simulink model "nonlinear_closed_g"  (R2024a)
settings: Solver=VariableStepAuto  StartTime=0.0  StopTime=30  MaxStep=1e-3  RelTol=1e-3
values from neighbouring files (symbols this model uses):
  A = [0, 1, 0, 0 ... (first row only)    [t_51.m]    (also in t_52.m)
  B = [0; J/Meff; 0; -beta/Meff]    [t_51.m]    (also in t_52.m)
  beta = m * lc    (= 40.0551)    [t_51.m]    (also in t_52.m)
  g = 9.81    [t_51.m]    (also in t_52.m)
  G_g = zeros(p_g)    [t_52.m]
  J = (1/3)*m1*l^2 + m2*l^2    (= 62.720658)    [t_51.m]    (also in t_52.m)
  K = [-46.28, -233.21, -10984.45, -3688.10]    [t_51.m]    (also in t_52.m)
  K_g = (U_g - K * X_g)    [t_52.m]
  M = 658.36    [t_51.m]    (also in t_52.m)
  m = m1 + m2    (= 30.46)    [t_51.m]    (also in t_52.m)
  w_g0 = zeros(p_g, 1)    [t_52.m]
  x0 = [0.1; 0.2; 0.03; 0.12]    [t_51.m]    (also in t_52.m)
  Y_g = zeros(1, p_g)    [t_52.m]
settings Model: Creator=eva  LastModifiedBy=eva

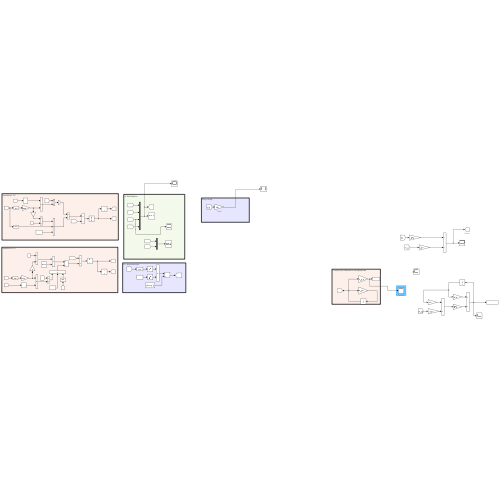
[thumbnail: Simulink's stored preview of the top-level diagram]
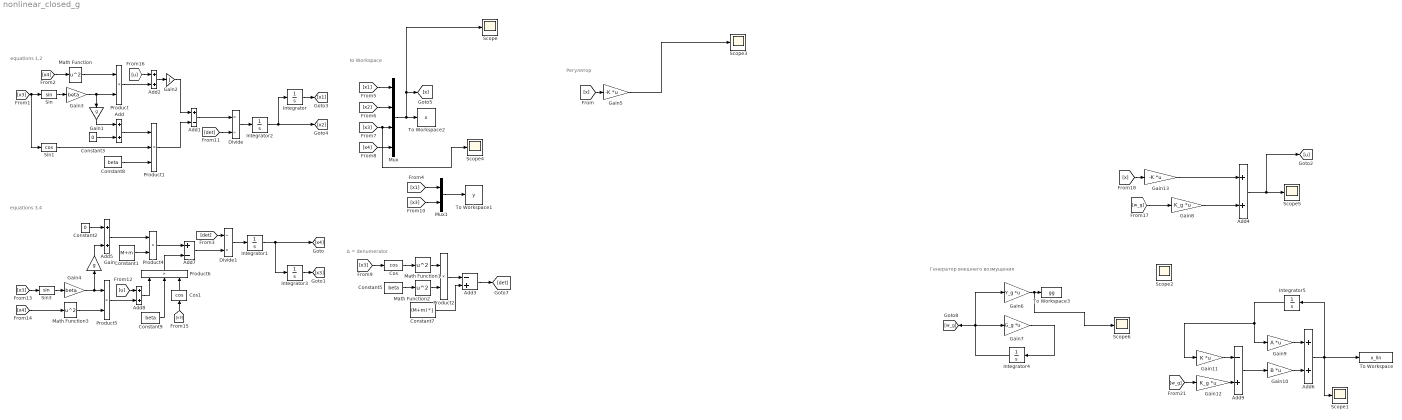
== system nonlinear_closed_g ==
  note: Регулятор
  note: to Workspace
  note: equations 1,2
  note: equations 3,4
  note: Δ = denumerator
  note: Генератор внешнего возмущения
  Add{,2,4..6,8} (6 alike) : Sum
  Add1 : Sum  Inputs=+-
  Add3 : Sum  Inputs=-+
  Add7 : Sum  Inputs=+-
  Add9 : Sum  Inputs=-+
  Constant1 : Constant  Value=M+m
  Constant2 : Constant  Value=0
  Constant3 : Constant  Value=0
  Constant5 : Constant  Value=beta
  Constant7 : Constant  Value=(M+m) * J
  Constant8 : Constant  Value=beta
  Constant9 : Constant  Value=beta
  Cos : Trigonometry  Operator=cos
  Cos1 : Trigonometry  Operator=cos
  Divide : Product  Inputs=*/
  Divide1 : Product  Inputs=/*
  Gain : Gain  Gain=g
  Gain1 : Gain  Gain=g
  Gain10 : Gain  Gain=B  Multiplication=Matrix(K*u)
  Gain11 : Gain  Gain=K  Multiplication=Matrix(K*u)
  Gain12 : Gain  Gain=K_g  Multiplication=Matrix(K*u)
  Gain13 : Gain  Gain=-K  Multiplication=Matrix(K*u)
  Gain2 : Gain  Gain=J
  Gain3 : Gain  Gain=beta
  Gain4 : Gain  Gain=beta
  Gain5 : Gain  Gain=-K  Multiplication=Matrix(K*u)
  Gain6 : Gain  Gain=Y_g  Multiplication=Matrix(K*u)
  Gain7 : Gain  Gain=G_g  Multiplication=Matrix(K*u)
  Gain8 : Gain  Gain=K_g  Multiplication=Matrix(K*u)
  Gain9 : Gain  Gain=A  Multiplication=Matrix(K*u)
  Integrator : Integrator  InitialCondition=x0(1)
  Integrator1 : Integrator  InitialCondition=x0(4)
  Integrator2 : Integrator  InitialCondition=x0(2)
  Integrator3 : Integrator  InitialCondition=x0(3)
  Integrator4 : Integrator  InitialCondition=w_g0
  Integrator5 : Integrator  InitialCondition=x0
  Math Function{,1..3} (4 alike) : Math  Operator=square
  Mux : Mux
  Mux1 : Mux  Inputs=2
  Product{,2,4..5} (4 alike) : Product
  Product1 : Product  Inputs=3
  Product6 : Product  Inputs=3
  Scope{,1..6} (7 alike) : Scope
  Sin : Trigonometry
  Sin1 : Trigonometry  Operator=cos
  Sin3 : Trigonometry
  To Workspace : ToWorkspace  VariableName=x_lin  SaveFormat=Structure With Time  SampleTime=-1
  To Workspace1 : ToWorkspace  VariableName=y  SaveFormat=Structure With Time  SampleTime=-1
  To Workspace2 : ToWorkspace  VariableName=x  SaveFormat=Structure With Time  SampleTime=-1
  To Workspace3 : ToWorkspace  VariableName=gg  SaveFormat=Structure With Time  SampleTime=-1
  wires:
  Divide/1 -> Integrator2/1
  Mux1/1 -> To Workspace1/1
  [x3] -> Mux1/2
  Gain3/1 -> Product/2, Gain1/1
  Sin/1 -> Gain3/1
  Mux/1 -> Scope/1, [x], To Workspace2/1
  Divide1/1 -> Integrator1/1
  Integrator2/1 -> [x2], Integrator/1
  Math Function3/1 -> Product5/2
  Constant8/1 -> Product1/3
  Math Function/1 -> Product/1
  [x4] -> Math Function/1
  [det] -> Divide/2
  [u] -> Add2/1
  Gain2/1 -> Add1/1
  Add/1 -> Product1/1
  [x3] -> Cos/1
  Math Function2/1 -> Product2/2
  Product4/1 -> Add7/1
  Constant3/1 -> Add/2
  Add2/1 -> Gain2/1
  [x3] -> Cos1/1
  [u] -> Add8/1
  Constant7/1 -> Add3/2
  Cos1/1 -> Product6/3
  [det] -> Divide1/1
  Constant9/1 -> Product6/2
  Math Function1/1 -> Product2/1
  [x3] -> Sin/1, Sin1/1
  [x4] -> Math Function3/1
  Product2/1 -> Add3/1
  Add8/1 -> Product6/1
  Integrator1/1 -> [x4], Integrator3/1
  Product5/1 -> Add8/2
  [x4] -> Mux/4
  [x3] -> Sin3/1
  Sin1/1 -> Product1/2
  Constant2/1 -> Add5/1
  Sin3/1 -> Gain4/1
  [x1] -> Mux/1
  Gain1/1 -> Add/1
  Gain/1 -> Add5/2
  Product6/1 -> Add7/2
  [x1] -> Mux1/1
  [x3] -> Scope4/1, Mux/3
  [x2] -> Mux/2
  Add7/1 -> Divide1/2
  Add3/1 -> [det]
  Integrator/1 -> [x1]
  Add1/1 -> Divide/1
  Product/1 -> Add2/2
  Constant5/1 -> Math Function2/1
  Gain5/1 -> Scope3/1
  Product1/1 -> Add1/2
  Gain4/1 -> Product5/1, Gain/1
  Integrator3/1 -> [x3]
  Cos/1 -> Math Function1/1
  Constant1/1 -> Product4/2
  Add5/1 -> Product4/1
  [x] -> Gain5/1
  Integrator4/1 -> [w_g], Gain7/1, Gain6/1
  [w_g] -> Gain12/1
  Gain9/1 -> Add6/1
  Gain6/1 -> Scope6/1, To Workspace3/1
  Gain10/1 -> Add6/2
  Add9/1 -> Gain10/1
  Gain12/1 -> Add9/2
  Integrator5/1 -> Gain9/1, Gain11/1
  Gain7/1 -> Integrator4/1
  [w_g] -> Gain8/1
  Add6/1 -> Scope1/1, To Workspace/1, Integrator5/1
  Gain11/1 -> Add9/1
  Gain8/1 -> Add4/2
  Gain13/1 -> Add4/1
  [x] -> Gain13/1
  Add4/1 -> [u], Scope5/1
